simulink model "siren"  (R2020a)
settings: Solver=VariableStepAuto  StartTime=0.0  StopTime=10.0  RelTol=1e-3
model workspace (MAT data in the model file):
  conflict_matrix = [0 1 1 0]
values from neighbouring files (symbols this model uses):
  amber_time_vector = [3 3]    [simple_intersection.m]    (also in variables.m)
  green_interval_matrix = [[0 5] [5 0]]    [simple_intersection.m]    (also in variables.m)
  yellow_time_vector = [3 3]    [simple_intersection.m]    (also in variables.m)
undefined symbols (not defined in the file or in its folder): num_lights
libraries: mpclib x1
settings Model: Creator=frede  LastModifiedBy=zinoex

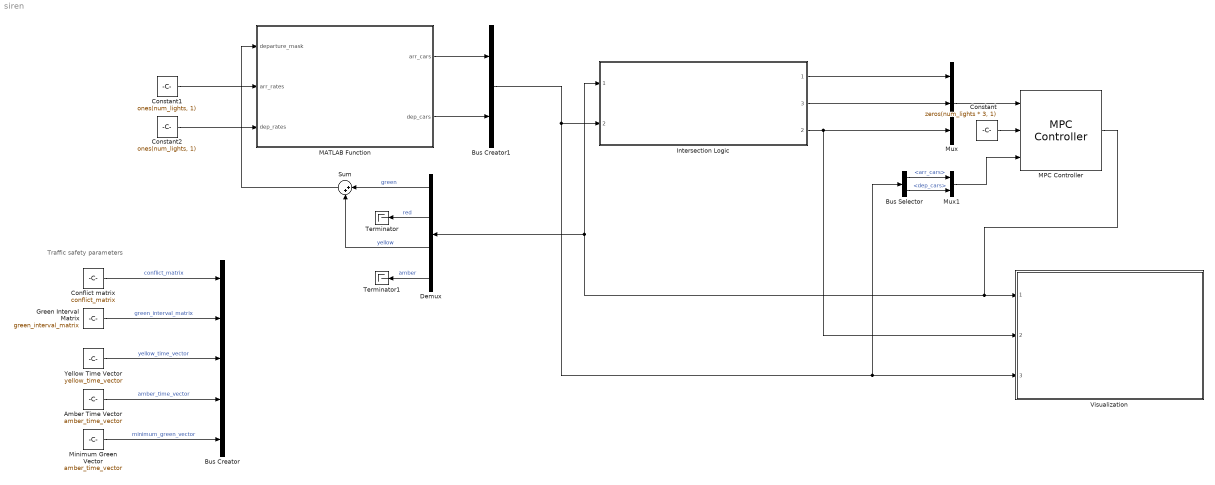
== system siren ==
  note: Traffic safety parameters
  Amber Time Vector : Constant  Value=amber_time_vector  VectorParams1D=off
  Bus Creator : BusCreator  Inputs=5
  Bus Creator1 : BusCreator  Inputs=2
  Bus Selector : BusSelector  OutputSignals=arr_cars,dep_cars
  Conflict matrix : Constant  Value=conflict_matrix  VectorParams1D=off
  Constant : Constant  Value=zeros(num_lights * 3, 1)  VectorParams1D=off
  Constant1 : Constant  Value=ones(num_lights, 1)  VectorParams1D=off
  Constant2 : Constant  Value=ones(num_lights, 1)
  Demux : Demux
  Green Interval Matrix : Constant  Value=green_interval_matrix  VectorParams1D=off
  Intersection Logic : Subsystem  ReferencedSubsystem=IntersectionLogic
      settings: PortSchema="{\"entries\":[{\"content\":{\"sides\":[{\"content\":{\"connectorIds\":[\"In1\",\"In2\"]},\"type\":\"ConnectorPlacement.EquallySpacedRectSide\",\"uuid\":\"6e6446de-a25b-4534-8ded-cf336778c054\"},{\"content\":{\"connectorIds\":[\"Out1\",\"Out3\",\"Out2\"],\"side\":\"RIGHT\"},\"type\":\"ConnectorPlacement.EquallySpacedRectSide\",\"uuid\":\"5658d63c-3b18-4ccf-b93a-8cba65e570bd\"},{\"content\":{\"connectorIds\":[],\"side\":\"TOP\"},\"type\":\"ConnectorPlacement.EquallySpacedRectSide\",\"uuid\":\"6d40bcf6-e3cf-4826-9a83-05e24177dc3c\"},{\"content\":{\"connectorIds\":[],\"side\":\"BOTTOM\"},\"type\":\"ConnectorPlacement.EquallySpacedRectSide\",\"uuid\":\"744b32b3-ee37-40a1-96d5-75305a689d6c\"}]},\"type\":\"ConnectorPlacement.EquallySpacedConnector\",\"uuid\":\"b3181e58-c706-47f0-8ee3-902276b1e437\"}],\"packageUris\":[\"http://schema.mathworks.com/mf0/Connector/19700101\"],\"version\":\"1.0\"}"
  MATLAB Function : MATLAB Function  TreatAsAtomicUnit=on
  MPC Controller : mpclib/MPC Controller  SCDEnableBlockLinearizationSpecification=on  is_multiple=0  enable_value=0  return_u0=off  updateMPCinCallerWorkspace=on  md_inport=on  mv_inport=off  uref_inport=off  return_cost=off  return_mvseq=off  return_qpstatus=off  return_xseq=off  return_state=off  return_ovseq=off  state_inport=off  umin_inport=off  umax_inport=off  ymin_inport=off  ymax_inport=off  cc_inport=off  ywt_inport=off  uwt_inport=off  duwt_inport=off  rhoeps_inport=off  pm_inport=off  MaximumP=10  HorizonChoice=FixedHorizon  n_ts=1  n_p=10  n_mv=4 * num_lights  n_md=2 * num_lights  n_ud=0  n_mo=3 * num_lights  n_uo=0  BlockDataType=double  SampleTimeInherited=off  switch_inport=off
  Minimum Green Vector : Constant  Value=amber_time_vector  VectorParams1D=off
  Mux : Mux  Inputs=3
  Mux1 : Mux  Inputs=2
  Sum : Sum  Inputs=|++
  Terminator : Terminator
  Terminator1 : Terminator
  Visualization : Subsystem  ReferencedSubsystem=Visualization
  Yellow Time Vector : Constant  Value=yellow_time_vector  VectorParams1D=off
  wires:
  Conflict matrix/1 -> Bus Creator/1  "conflict_matrix"
  Green Interval Matrix/1 -> Bus Creator/2  "green_interval_matrix"
  Yellow Time Vector/1 -> Bus Creator/3  "yellow_time_vector"
  Amber Time Vector/1 -> Bus Creator/4  "amber_time_vector"
  Minimum Green Vector/1 -> Bus Creator/5  "minimum_green_vector"
  Intersection Logic/3 -> Mux/2
  Mux/1 -> MPC Controller/1
  Constant/1 -> MPC Controller/2
  MATLAB Function/1(arr_cars) -> Bus Creator1/1
  MATLAB Function/2(dep_cars) -> Bus Creator1/2
  Constant1/1 -> MATLAB Function/2(arr_rates)
  Constant2/1 -> MATLAB Function/3(dep_rates)
  Bus Creator1/1 -> Bus Selector/1, Visualization/3, Intersection Logic/2
  Mux1/1 -> MPC Controller/3
  Bus Selector/1 -> Mux1/1  "<arr_cars>"
  Bus Selector/2 -> Mux1/2  "<dep_cars>"
  MPC Controller/1 -> Demux/1, Intersection Logic/1, Visualization/1
  Intersection Logic/1 -> Mux/1
  Intersection Logic/2 -> Mux/3, Visualization/2
  Demux/1 -> Sum/1  "green"
  Demux/3 -> Sum/2  "yellow"
  Sum/1 -> MATLAB Function/1(departure_mask)
  Demux/2 -> Terminator/1  "red"
  Demux/4 -> Terminator1/1  "amber"

== matlab function siren/MATLAB Function ==
  data: departure_mask input; arr_cars output; arr_rates input; dep_rates input; dep_cars output
function [arr_cars, dep_cars] = simulate_traffic(departure_mask, arr_rates, dep_rates)
% Uses Poisson Distribution to simulate cars arriving and departing intersection
%     Inputs:
%         colors - column vector of boolean values representing the light in each lane
%         arr_rates, dep_rates - arrival and departure rates of cars (for each lane)
%             **Rates should be specified with units of cars/timestep
%     Outputs:
%           arr_cars, dep_cars - number of cars arriving and departing each
%           lane (whole numbers)
    arr_cars = poissrnd(arr_rates);
    dep_cars = poissrnd(dep_rates) .* departure_mask;
